simulink library "ESTS_FRIC_SLIP"  (R2024b)
settings: Solver=VariableStepAuto  StartTime=0.0  StopTime=10.0  RelTol=1e-3
undefined symbols (not defined in the file): ESTS_FRIC_p1_MovAvgCoef_na, ESTS_FRIC_p_TirSatLim_na, ESTS_FRIC_SLIP_p_SwtFriMet_na
libraries: VUT_lib x4, simulink x1
settings Model: Creator=blatak  LastModifiedBy=blatak

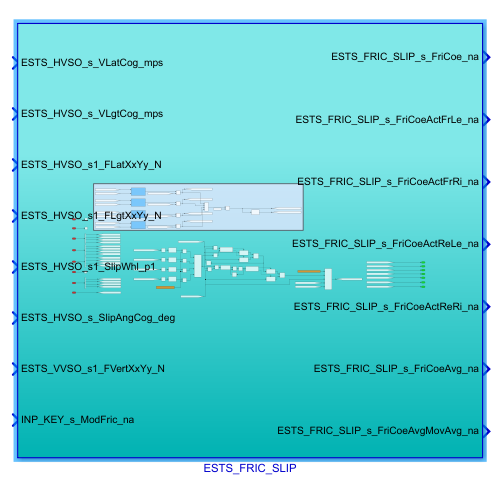
[thumbnail: Simulink's stored preview of the top-level diagram]
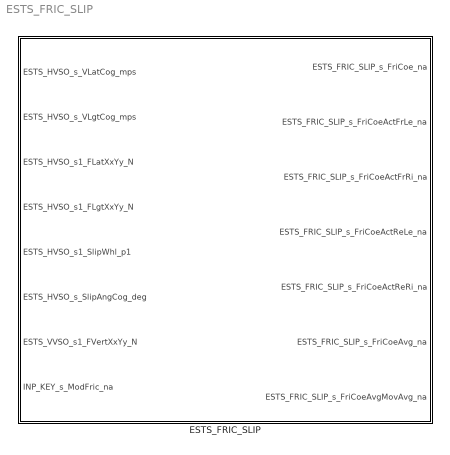
== system ESTS_FRIC_SLIP ==
  ESTS_FRIC_SLIP : Subsystem

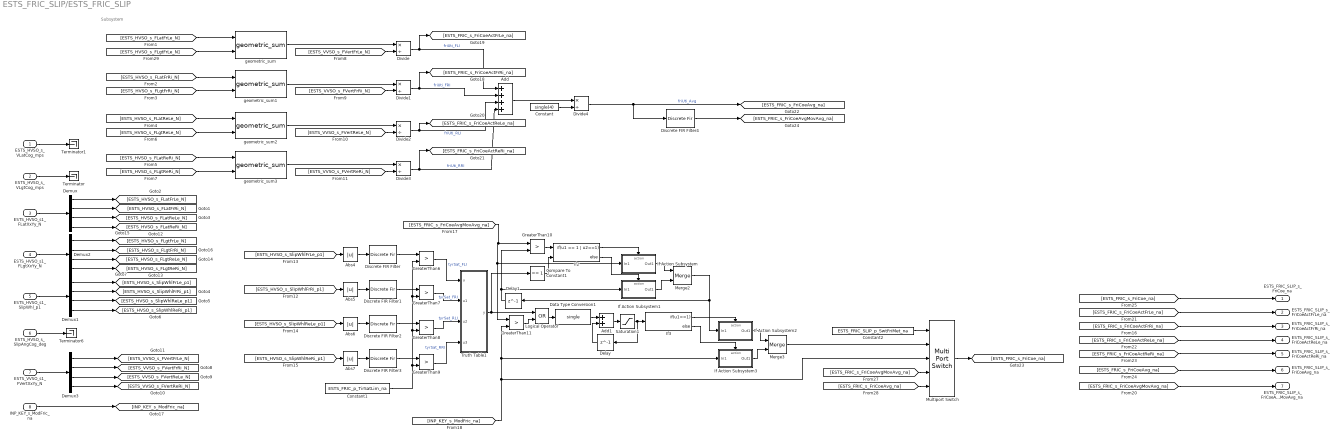
== system ESTS_FRIC_SLIP/ESTS_FRIC_SLIP ==
  note: Subsystem
  ESTS_HVSO_s_VLatCog_mps : Inport
  ESTS_HVSO_s_VLgtCog_mps : Inport  Port=2
  ESTS_HVSO_s1_FLatXxYy_N : Inport  Port=3
  ESTS_HVSO_s1_FLgtXxYy_N : Inport  Port=4
  ESTS_HVSO_s1_SlipWhl_p1 : Inport  Port=5
  ESTS_HVSO_s_SlipAngCog_deg : Inport  Port=6
  ESTS_VVSO_s1_FVertXxYy_N : Inport  Port=7
  INP_KEY_s_ModFric_na : Inport  Port=8
  Abs{4..7} (4 alike) : Abs  SaturateOnIntegerOverflow=off
  Add : Sum  Inputs=++++
  Add1 : Sum
  Compare To Constant1 : simulink/Logic and Bit Operations/Compare To Constant  relop===  const=1  OutDataTypeStr=boolean
  Constant : Constant  Value=single(4)
  Constant1 : Constant  Value=ESTS_FRIC_p_TirSatLim_na
  Constant2 : Constant  Value=ESTS_FRIC_SLIP_p_SwtFriMet_na
  Data Type Conversion1 : DataTypeConversion  OutDataTypeStr=single  SaturateOnIntegerOverflow=off  RndMeth=Floor
  Delay : Delay  DelayLength=1
  Delay1 : Delay  DelayLength=1
  Demux{,1..3} (4 alike) : Demux
  Discrete FIR Filter{,1..4} (5 alike) : DiscreteFir  Coefficients=ESTS_FRIC_p1_MovAvgCoef_na
  Divide{,1..4} (5 alike) : Product  Inputs=*/
  GreaterThan{6..11} (6 alike) : RelationalOperator  Operator=>  OutDataTypeStr=boolean  RndMeth=Simplest  InputSameDT=off
  If Action Subsystem : Subsystem  TreatAsAtomicUnit=on
  If Action Subsystem1 : Subsystem  TreatAsAtomicUnit=on
  If Action Subsystem2 : Subsystem  TreatAsAtomicUnit=on
  If Action Subsystem3 : Subsystem  TreatAsAtomicUnit=on
  If2 : If  NumInputs=2  IfExpression=u1 == 1 | u2==1
  If3 : If  IfExpression=u1==1
  Logical Operator : Logic  Operator=OR  AllPortsSameDT=off  OutDataTypeStr=boolean
  Merge2 : Merge
  Merge3 : Merge
  Multiport Switch : MultiPortSwitch  Inputs=4  SaturateOnIntegerOverflow=off  InputSameDT=off
  Saturation1 : Saturate  UpperLimit=1  LowerLimit=0
  Terminator : Terminator
  Terminator1 : Terminator
  Terminator6 : Terminator
  Truth Table1 : Truth Table  TreatAsAtomicUnit=on
  geometric_sum{,1..3} (4 alike) : VUT_lib/geometric_sum  SystemSampleTime=-1  VariantActivationTime=update diagram  AllowFlexibleInterface=on  Latency=0  AutoFrameSizeCalculation=off
  ESTS_FRIC_SLIP_s_FriCoe_na : Outport
  ESTS_FRIC_SLIP_s_FriCoeActFrLe_na : Outport  Port=2
  ESTS_FRIC_SLIP_s_FriCoeActFrRi_na : Outport  Port=3
  ESTS_FRIC_SLIP_s_FriCoeActReLe_na : Outport  Port=4
  ESTS_FRIC_SLIP_s_FriCoeActReRi_na : Outport  Port=5
  ESTS_FRIC_SLIP_s_FriCoeAvg_na : Outport  Port=6
  ESTS_FRIC_SLIP_s_FriCoeAvgMovAvg_na : Outport  Port=7
  wires:
  [ESTS_FRIC_s_FriCoeActFrLe_na] -> ESTS_FRIC_SLIP_s_FriCoeActFrLe_na/1
  [ESTS_FRIC_s_FriCoeActReRi_na] -> ESTS_FRIC_SLIP_s_FriCoeActReRi_na/1
  ESTS_HVSO_s1_SlipWhl_p1/1 -> Demux1/1
  ESTS_HVSO_s_SlipAngCog_deg/1 -> Terminator6/1
  Discrete FIR Filter1/1 -> GreaterThan7/1
  Divide3/1 -> [ESTS_FRIC_s_FriCoeActReRi_na], Add/4  "friUti_RRI"
  Divide4/1 -> [ESTS_FRIC_s_FriCoeAvg_na], Discrete FIR Filter4/1  "friUti_Avg"
  If Action Subsystem/1(Out1) -> Merge2/1
  GreaterThan9/1 -> Truth Table1/4(u3)  "tyrSat_RRI"
  Merge2/1 -> If Action Subsystem2/1(In1), Delay1/1
  Demux3/2 -> [ESTS_VVSO_s_FVertFrRi_N]
  [ESTS_FRIC_s_FriCoeActReLe_na] -> ESTS_FRIC_SLIP_s_FriCoeActReLe_na/1
  [ESTS_HVSO_s_SlipWhlReRi_p1] -> Abs7/1
  If Action Subsystem2/1(Out1) -> Merge3/1
  Divide1/1 -> [ESTS_FRIC_s_FriCoeActFrRi_na], Add/2  "friUti_FRI"
  [ESTS_FRIC_s_FriCoeAvgMovAvg_na] -> Multiport Switch/4
  Merge3/1 -> Multiport Switch/2
  geometric_sum1/1 -> Divide1/1
  If2/2 -> If Action Subsystem1/Action
  [ESTS_FRIC_s_FriCoeAvgMovAvg_na] -> GreaterThan10/1, If Action Subsystem/1(In1), GreaterThan11/1
  If2/1 -> If Action Subsystem/Action
  Truth Table1/1(y) -> Logical Operator/1, Compare To Constant1/1
  Demux1/1 -> [ESTS_HVSO_s_SlipWhlFrLe_p1]
  geometric_sum3/1 -> Divide3/1
  [ESTS_VVSO_s_FVertFrRi_N] -> Divide1/2
  Demux2/2 -> [ESTS_HVSO_s_FLgtFrRi_N]
  Add1/1 -> Saturation1/1
  [ESTS_FRIC_s_FriCoeAvg_na] -> ESTS_FRIC_SLIP_s_FriCoeAvg_na/1
  If3/1 -> If Action Subsystem2/Action
  Constant1/1 -> GreaterThan9/2, GreaterThan8/2, GreaterThan7/2, GreaterThan6/2
  [ESTS_FRIC_s_FriCoeAvgMovAvg_na] -> ESTS_FRIC_SLIP_s_FriCoeAvgMovAvg_na/1
  Demux/4 -> [ESTS_HVSO_s_FLatReRi_N]
  Discrete FIR Filter4/1 -> [ESTS_FRIC_s_FriCoeAvgMovAvg_na]
  [ESTS_HVSO_s_FLgtFrLe_N] -> geometric_sum/2
  GreaterThan10/1 -> If2/1
  ESTS_VVSO_s1_FVertXxYy_N/1 -> Demux3/1
  Discrete FIR Filter3/1 -> GreaterThan9/1
  Abs6/1 -> Discrete FIR Filter2/1
  [ESTS_HVSO_s_SlipWhlReLe_p1] -> Abs6/1
  [ESTS_HVSO_s_FLgtReRi_N] -> geometric_sum3/2
  geometric_sum2/1 -> Divide2/1
  Demux/2 -> [ESTS_HVSO_s_FLatFrRi_N]
  If Action Subsystem3/1(Out1) -> Merge3/2
  Data Type Conversion1/1 -> Add1/1
  Add/1 -> Divide4/1
  GreaterThan11/1 -> Logical Operator/2
  [ESTS_VVSO_s_FVertReRi_N] -> Divide3/2
  Demux3/4 -> [ESTS_VVSO_s_FVertReRi_N]
  [ESTS_HVSO_s_FLatFrLe_N] -> geometric_sum/1
  Saturation1/1 -> Delay/1, If3/1
  Discrete FIR Filter2/1 -> GreaterThan8/1
  Logical Operator/1 -> Data Type Conversion1/1
  ESTS_HVSO_s_VLgtCog_mps/1 -> Terminator/1
  Abs7/1 -> Discrete FIR Filter3/1
  ESTS_HVSO_s_VLatCog_mps/1 -> Terminator1/1
  [ESTS_VVSO_s_FVertFrLe_N] -> Divide/2
  Constant/1 -> Divide4/2
  [ESTS_HVSO_s_SlipWhlFrRi_p1] -> Abs5/1
  Demux1/2 -> [ESTS_HVSO_s_SlipWhlFrRi_p1]
  [ESTS_HVSO_s_FLgtFrRi_N] -> geometric_sum1/2
  Multiport Switch/1 -> [ESTS_FRIC_s_FriCoe_na]
  [ESTS_VVSO_s_FVertReLe_N] -> Divide2/2
  Demux/1 -> [ESTS_HVSO_s_FLatFrLe_N]
  GreaterThan8/1 -> Truth Table1/3(u2)  "tyrSat_RLI"
  Demux/3 -> [ESTS_HVSO_s_FLatReLe_N]
  geometric_sum/1 -> Divide/1
  [ESTS_HVSO_s_FLatReRi_N] -> geometric_sum3/1
  [INP_KEY_s_ModFric_na] -> Multiport Switch/3, If Action Subsystem3/1(In1), GreaterThan11/2
  Discrete FIR Filter/1 -> GreaterThan6/1
  Abs4/1 -> Discrete FIR Filter/1
  Demux2/4 -> [ESTS_HVSO_s_FLgtReRi_N]
  Demux3/1 -> [ESTS_VVSO_s_FVertFrLe_N]
  Delay/1 -> Add1/2
  Abs5/1 -> Discrete FIR Filter1/1
  [ESTS_HVSO_s_FLgtReLe_N] -> geometric_sum2/2
  ESTS_HVSO_s1_FLgtXxYy_N/1 -> Demux2/1
  If Action Subsystem1/1(Out1) -> Merge2/2
  [ESTS_FRIC_s_FriCoeAvg_na] -> Multiport Switch/5
  Demux1/3 -> [ESTS_HVSO_s_SlipWhlReLe_p1]
  [ESTS_HVSO_s_FLatFrRi_N] -> geometric_sum1/1
  ESTS_HVSO_s1_FLatXxYy_N/1 -> Demux/1
  GreaterThan7/1 -> Truth Table1/2(u1)  "tyrSat_FRI"
  [ESTS_FRIC_s_FriCoeActFrRi_na] -> ESTS_FRIC_SLIP_s_FriCoeActFrRi_na/1
  Demux3/3 -> [ESTS_VVSO_s_FVertReLe_N]
  [ESTS_FRIC_s_FriCoe_na] -> ESTS_FRIC_SLIP_s_FriCoe_na/1
  Demux2/3 -> [ESTS_HVSO_s_FLgtReLe_N]
  INP_KEY_s_ModFric_na/1 -> [INP_KEY_s_ModFric_na]
  Delay1/1 -> If Action Subsystem1/1(In1), GreaterThan10/2
  Divide/1 -> Add/1, [ESTS_FRIC_s_FriCoeActFrLe_na]  "friUti_FLI"
  If3/2 -> If Action Subsystem3/Action
  [ESTS_HVSO_s_SlipWhlFrLe_p1] -> Abs4/1
  GreaterThan6/1 -> Truth Table1/1(u)  "tyrSat_FLI"
  Demux2/1 -> [ESTS_HVSO_s_FLgtFrLe_N]
  Divide2/1 -> [ESTS_FRIC_s_FriCoeActReLe_na], Add/3  "friUti_RLI"
  Compare To Constant1/1 -> If2/2
  [ESTS_HVSO_s_FLatReLe_N] -> geometric_sum2/1
  Demux1/4 -> [ESTS_HVSO_s_SlipWhlReRi_p1]
  Constant2/1 -> Multiport Switch/1

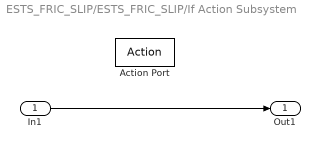
== system ESTS_FRIC_SLIP/ESTS_FRIC_SLIP/If Action Subsystem ==
  In1 : Inport
  Action Port : ActionPort  ActionPortLabel=if(u1 == 1 | u2==1)
  Out1 : Outport
  wires:
  In1/1 -> Out1/1

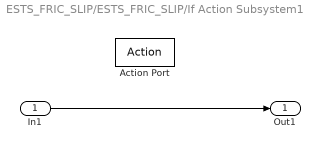
== system ESTS_FRIC_SLIP/ESTS_FRIC_SLIP/If Action Subsystem1 ==
  In1 : Inport
  Action Port : ActionPort  ActionPortLabel=else
  Out1 : Outport
  wires:
  In1/1 -> Out1/1

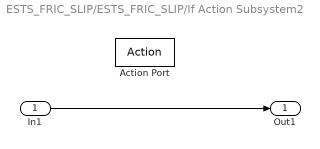
== system ESTS_FRIC_SLIP/ESTS_FRIC_SLIP/If Action Subsystem2 ==
  In1 : Inport
  Action Port : ActionPort  ActionPortLabel=if(u1==1)
  Out1 : Outport
  wires:
  In1/1 -> Out1/1

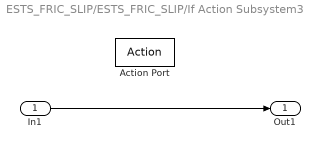
== system ESTS_FRIC_SLIP/ESTS_FRIC_SLIP/If Action Subsystem3 ==
  In1 : Inport
  Action Port : ActionPort  ActionPortLabel=else
  Out1 : Outport
  wires:
  In1/1 -> Out1/1

== matlab function ESTS_FRIC_SLIP/Truth Table1 ==
  data: u input; y output single; u1 input; u2 input; u3 input
function y = fcn(u, u1, u2, u3)

aVarTruthTableCondition_1 = false;
aVarTruthTableCondition_2 = false;
aVarTruthTableCondition_3 = false;
aVarTruthTableCondition_4 = false;


% Example condition 1

aVarTruthTableCondition_1 = logical(u == 1);

% Example condition 2

aVarTruthTableCondition_2 = logical(u1 == 1);

% Example condition 3

aVarTruthTableCondition_3 = logical(u2 == 1);

% Example condition 4

aVarTruthTableCondition_4 = logical(u3 == 1);

if (aVarTruthTableCondition_1 && aVarTruthTableCondition_2)
    aFcnTruthTableAction_1();
elseif (aVarTruthTableCondition_1 && aVarTruthTableCondition_3)
    aFcnTruthTableAction_1();
elseif (aVarTruthTableCondition_1 && aVarTruthTableCondition_4)
    aFcnTruthTableAction_1();
elseif (aVarTruthTableCondition_2 && aVarTruthTableCondition_3)
    aFcnTruthTableAction_1();
elseif (aVarTruthTableCondition_2 && aVarTruthTableCondition_4)
    aFcnTruthTableAction_1();
elseif (aVarTruthTableCondition_3 && aVarTruthTableCondition_4)
    aFcnTruthTableAction_1();
elseif (~aVarTruthTableCondition_1 && ~aVarTruthTableCondition_2 && ~aVarTruthTableCondition_3)
    aFcnTruthTableAction_2();
elseif (~aVarTruthTableCondition_1 && ~aVarTruthTableCondition_3 && ~aVarTruthTableCondition_4)
    aFcnTruthTableAction_2();
elseif (~aVarTruthTableCondition_1 && ~aVarTruthTableCondition_2 && ~aVarTruthTableCondition_4)
    aFcnTruthTableAction_2();
else % Default
    aFcnTruthTableAction_2();
end

function aFcnTruthTableAction_1()

% Example action 1 called from D1 & D2 column in condition table

y = 1;

function aFcnTruthTableAction_2()

% Example action 2 called from D3 column in condition table

y = 0;
